simulink model "LA_3b"  (R2021a)
settings: Solver=VariableStepAuto  StartTime=0.0  StopTime=10.0  RelTol=1e-3
model workspace (MAT data in the model file):
  G = 5395.5
  Kpv = 25
  Kpx = 2
  T_m = 0.2
  g = 9.81
  k_m = 100
  m = 550
  m_G = 450
libraries: Regler x7, AnimationenLib x1
settings Model: OrderedModelArguments=off  Creator=Manoli  LastModifiedBy=Manoli

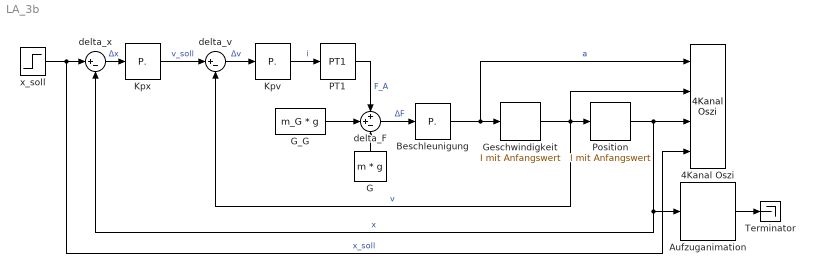
== system LA_3b ==
  " delta_F" : Sum  Inputs=++-  InputSameDT=on  SaturateOnIntegerOverflow=on  OutDataTypeStr=Inherit: Same as first input
  4Kanal Oszi : Regler/4Kanal Oszi  N=20000  k=[1 1 1 1]  y=[-5 5]  tmax=1
  Aufzuganimation : AnimationenLib/Aufzuganimation  T=0.1
  Beschleunigung : Regler/P.  k=1/(m + m_G)
  G : Constant  Value=m * g
  G_G : Constant  Value=m_G * g
  Geschwindigkeit : Regler/I mit Anfangswert  Ti=1  u0=0
  Kpv : Regler/P.  k=Kpv
  Kpx : Regler/P.  k=Kpx
  PT1 : Regler/PT1  k=k_m  T1=T_m
  Position : Regler/I mit Anfangswert  Ti=1  u0=10
  Terminator : Terminator
  delta_v : Sum  Inputs=|+-  InputSameDT=on  SaturateOnIntegerOverflow=on  OutDataTypeStr=Inherit: Same as first input
  delta_x : Sum  Inputs=|+-  InputSameDT=on  SaturateOnIntegerOverflow=on  OutDataTypeStr=Inherit: Same as first input
  x_soll : Step  Time=0.000001  Before=10  After=16  SampleTime=0
  wires:
  Geschwindigkeit/1 -> delta_v/2, 4Kanal Oszi/2, Position/1  "v"
  Position/1 -> Aufzuganimation/1, delta_x/2, 4Kanal Oszi/3  "x"
  " delta_F"/1 -> Beschleunigung/1  "ΔF"
  G/1 -> " delta_F"/3
  G_G/1 -> " delta_F"/2
  PT1/1 -> " delta_F"/1  "F_A"
  Beschleunigung/1 -> Geschwindigkeit/1, 4Kanal Oszi/1  "a"
  x_soll/1 -> delta_x/1, 4Kanal Oszi/4  "x_soll"
  delta_v/1 -> Kpv/1  "Δv"
  Kpv/1 -> PT1/1  "i"
  delta_x/1 -> Kpx/1  "Δx"
  Kpx/1 -> delta_v/1  "v_soll"
  Aufzuganimation/1 -> Terminator/1
